simulink library "dlbsBlockExtractGradientGF"  (R2025b)
settings: Solver=VariableStepAuto  StartTime=0.0  StopTime=10.0  RelTol=1e-3
settings Model: Creator=lt6037  LastModifiedBy=lt6037

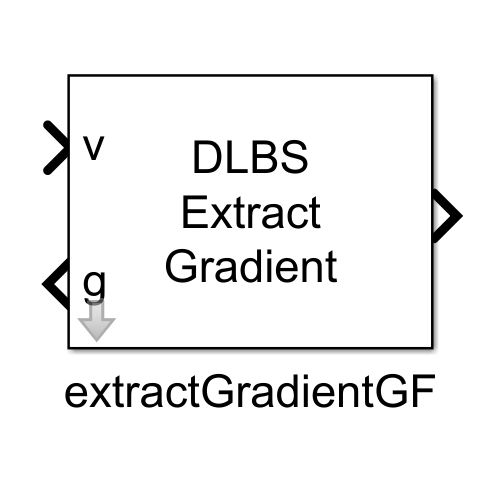
[thumbnail: Simulink's stored preview of the top-level diagram]
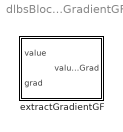
== system dlbsBlockExtractGradientGF ==
  extractGradientGF : Subsystem
      settings: PortSchema="{\"entries\":[{\"content\":{\"sides\":[{\"content\":{\"connectorIds\":[\"In1\",\"Out2\"]},\"type\":\"ConnectorPlacement.EquallySpacedRectSide\",\"uuid\":\"d7bd6d00-f861-4c9f-9c86-2de2a827f2a5\"},{\"content\":{\"connectorIds\":[\"Out1\"],\"side\":\"RIGHT\"},\"type\":\"ConnectorPlacement.EquallySpacedRectSide\",\"uuid\":\"6c6147b6-7369-4ee4-b487-1b85ba929b69\"},{\"content\":{\"side\":\"TOP\"},\"type\":\"ConnectorPlacement.EquallySpacedRectSide\",\"uuid\":\"81f8b5ae-e1d6-45a0-9bd6-89f53e78f0c4\"}]},\"type\":\"ConnectorPlacement.EquallySpacedConnector\",\"uuid\":\"2fcec617-149d-4efc-b95b-c44947a16900\"}],\"packageUris\":[\"http://schema.mathworks.com/mf0/Connector/R2020b\"],\"version\":\"1.0\"}"
      mask Display:
      | % val + grad
      | port_label('output', 1, '');
      | % grad
      | port_label('output', 2, 'g');
      | % val
      | port_label('input', 1, 'v');
      | disp("DLBS\nExtract\nGradient")

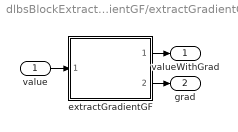
== system dlbsBlockExtractGradientGF/extractGradientGF ==
  value : Inport
  extractGradientGF : Subsystem  ReferencedSubsystem=dlbsSubsystemExtractGradientGF
  valueWithGrad : Outport
  grad : Outport  Port=2
  wires:
  extractGradientGF/2 -> grad/1
  value/1 -> extractGradientGF/1
  extractGradientGF/1 -> valueWithGrad/1
